simulink model "escooter_sequence_diagram_unlocking"  (R2025b)
settings: Solver=VariableStepAuto  StartTime=0.0  StopTime=10.0  RelTol=1e-3
settings Model: Creator=320236370  LastModifiedBy=320236370

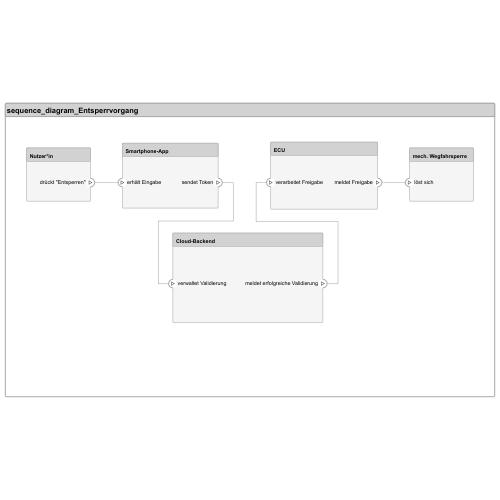
[thumbnail: Simulink's stored preview of the top-level diagram]
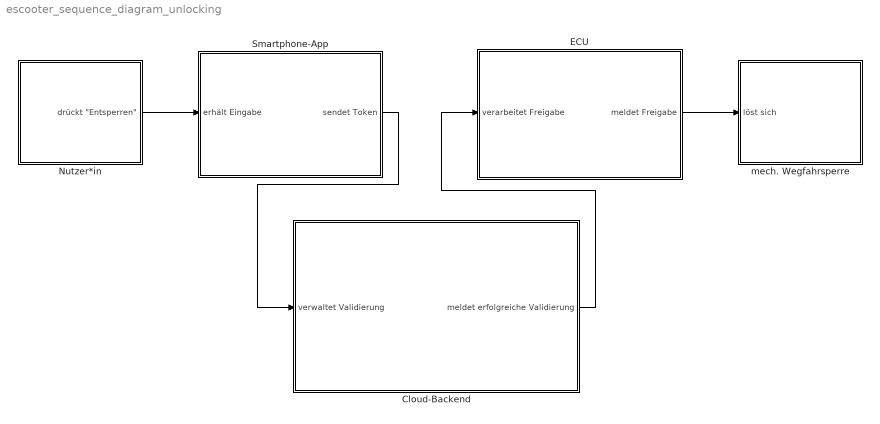
== system escooter_sequence_diagram_unlocking ==
  Cloud-Backend : Subsystem
      settings: PortSchema="{\"entries\":[{\"content\":{\"headerSize\":26,\"margin\":15,\"minimumSpacing\":25,\"sides\":[{\"content\":{\"connectorIds\":[\"In1\"]},\"type\":\"ConnectorPlacement.EquallySpacedRectSide\",\"uuid\":\"3d49029f-ff69-43f0-9083-eb7baed04898\"},{\"content\":{\"connectorIds\":[\"Out1\"],\"side\":\"RIGHT\"},\"type\":\"ConnectorPlacement.EquallySpacedRectSide\",\"uuid\":\"1597d90c-c332-40d9-8a70-68f04d256300\"},{\"content\":{\"side\":\"TOP\"},\"type\":\"ConnectorPlacement.EquallySpacedRectSide\",\"uuid\":\"ad895052-9fa6-4dfa-a28f-1843b80a8a3f\"},{\"content\":{\"side\":\"BOTTOM\"},\"type\":\"ConnectorPlacement.EquallySpacedRectSide\",\"uuid\":\"18bba2d1-49bf-4995-9855-eab6e9c91613\"}]},\"type\":\"ConnectorPlacement.EquallySpacedConnector\",\"uuid\":\"8d35fef0-5689-4d8b-850c-97501fa910c2\"}],\"packageUris\":[\"http://schema.mathworks.com/mf0/Connector/R2020b\"],\"version\":\"1.0\"}"
  ECU : Subsystem
      settings: PortSchema="{\"entries\":[{\"content\":{\"headerSize\":26,\"margin\":15,\"minimumSpacing\":25,\"sides\":[{\"content\":{\"connectorIds\":[\"In1\"]},\"type\":\"ConnectorPlacement.EquallySpacedRectSide\",\"uuid\":\"3d49029f-ff69-43f0-9083-eb7baed04898\"},{\"content\":{\"connectorIds\":[\"Out1\"],\"side\":\"RIGHT\"},\"type\":\"ConnectorPlacement.EquallySpacedRectSide\",\"uuid\":\"1597d90c-c332-40d9-8a70-68f04d256300\"},{\"content\":{\"side\":\"TOP\"},\"type\":\"ConnectorPlacement.EquallySpacedRectSide\",\"uuid\":\"ad895052-9fa6-4dfa-a28f-1843b80a8a3f\"}]},\"type\":\"ConnectorPlacement.EquallySpacedConnector\",\"uuid\":\"8d35fef0-5689-4d8b-850c-97501fa910c2\"}],\"packageUris\":[\"http://schema.mathworks.com/mf0/Connector/R2020b\"],\"version\":\"1.0\"}"
  Nutzer*in : Subsystem
      settings: PortSchema="{\"entries\":[{\"content\":{\"headerSize\":26,\"margin\":15,\"minimumSpacing\":25,\"sides\":[{\"content\":{},\"type\":\"ConnectorPlacement.EquallySpacedRectSide\",\"uuid\":\"3d49029f-ff69-43f0-9083-eb7baed04898\"},{\"content\":{\"connectorIds\":[\"Out1\"],\"side\":\"RIGHT\"},\"type\":\"ConnectorPlacement.EquallySpacedRectSide\",\"uuid\":\"1597d90c-c332-40d9-8a70-68f04d256300\"},{\"content\":{\"side\":\"TOP\"},\"type\":\"ConnectorPlacement.EquallySpacedRectSide\",\"uuid\":\"ad895052-9fa6-4dfa-a28f-1843b80a8a3f\"}]},\"type\":\"ConnectorPlacement.EquallySpacedConnector\",\"uuid\":\"8d35fef0-5689-4d8b-850c-97501fa910c2\"}],\"packageUris\":[\"http://schema.mathworks.com/mf0/Connector/R2020b\"],\"version\":\"1.0\"}"
  Smartphone-App : Subsystem
      settings: PortSchema="{\"entries\":[{\"content\":{\"headerSize\":26,\"margin\":15,\"minimumSpacing\":25,\"sides\":[{\"content\":{\"connectorIds\":[\"In1\"]},\"type\":\"ConnectorPlacement.EquallySpacedRectSide\",\"uuid\":\"3d49029f-ff69-43f0-9083-eb7baed04898\"},{\"content\":{\"connectorIds\":[\"Out1\"],\"side\":\"RIGHT\"},\"type\":\"ConnectorPlacement.EquallySpacedRectSide\",\"uuid\":\"1597d90c-c332-40d9-8a70-68f04d256300\"},{\"content\":{\"side\":\"TOP\"},\"type\":\"ConnectorPlacement.EquallySpacedRectSide\",\"uuid\":\"ad895052-9fa6-4dfa-a28f-1843b80a8a3f\"}]},\"type\":\"ConnectorPlacement.EquallySpacedConnector\",\"uuid\":\"8d35fef0-5689-4d8b-850c-97501fa910c2\"}],\"packageUris\":[\"http://schema.mathworks.com/mf0/Connector/R2020b\"],\"version\":\"1.0\"}"
  mech. Wegfahrsperre : Subsystem
      settings: PortSchema="{\"entries\":[{\"content\":{\"headerSize\":26,\"margin\":15,\"minimumSpacing\":25,\"sides\":[{\"content\":{\"connectorIds\":[\"In1\"]},\"type\":\"ConnectorPlacement.EquallySpacedRectSide\",\"uuid\":\"3d49029f-ff69-43f0-9083-eb7baed04898\"},{\"content\":{\"side\":\"RIGHT\"},\"type\":\"ConnectorPlacement.EquallySpacedRectSide\",\"uuid\":\"1597d90c-c332-40d9-8a70-68f04d256300\"},{\"content\":{\"side\":\"TOP\"},\"type\":\"ConnectorPlacement.EquallySpacedRectSide\",\"uuid\":\"ad895052-9fa6-4dfa-a28f-1843b80a8a3f\"}]},\"type\":\"ConnectorPlacement.EquallySpacedConnector\",\"uuid\":\"8d35fef0-5689-4d8b-850c-97501fa910c2\"}],\"packageUris\":[\"http://schema.mathworks.com/mf0/Connector/R2020b\"],\"version\":\"1.0\"}"
  wires:
  Nutzer*in/1("drückt \"Entsperren\"") -> Smartphone-App/1(erhält Eingabe)
  Smartphone-App/1(sendet Token) -> Cloud-Backend/1(verwaltet Validierung)
  Cloud-Backend/1(meldet erfolgreiche Validierung) -> ECU/1(verarbeitet Freigabe)
  ECU/1(meldet Freigabe) -> mech. Wegfahrsperre/1(löst sich)

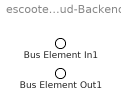
== system escooter_sequence_diagram_unlocking/Cloud-Backend ==
  Bus Element In1 : Inport  PortName=verwaltet Validierung
  Bus Element Out1 : Outport  PortName=meldet erfolgreiche Validierung

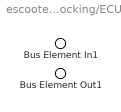
== system escooter_sequence_diagram_unlocking/ECU ==
  Bus Element In1 : Inport  PortName=verarbeitet Freigabe
  Bus Element Out1 : Outport  PortName=meldet Freigabe

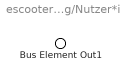
== system escooter_sequence_diagram_unlocking/Nutzer*in ==
  Bus Element Out1 : Outport  PortName="drückt \"Entsperren\""

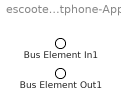
== system escooter_sequence_diagram_unlocking/Smartphone-App ==
  Bus Element In1 : Inport  PortName=erhält Eingabe
  Bus Element Out1 : Outport  PortName=sendet Token

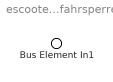
== system escooter_sequence_diagram_unlocking/mech. Wegfahrsperre ==
  Bus Element In1 : Inport  PortName=löst sich
